simulink model "fsm_12B_global"  (R2024b)
settings: Solver=FixedStepAuto  StartTime=0.0  StopTime=10  RelTol=1e-3
settings Model: Creator=elliocm  LastModifiedBy=lukeubun
settings SolverCC: AlgebraicLoopSolver=TrustRegion
settings DataIOCC: LimitDataPoints=on  SaveFormat=Array  ReturnWorkspaceOutputs=off
settings OptimizationCC: DefaultParameterBehavior=Inlined  UseDivisionForNetSlopeComputation=on  GainParamInheritBuiltInType=on  UseFloatMulNetSlope=on  InlineInvariantSignals=on  PassReuseOutputArgsAs=Individual arguments  ExpressionDepthLimit=2147483647  ZeroExternalMemoryAtStartup=off  ZeroInternalMemoryAtStartup=off  NoFixptDivByZeroProtection=on  EfficientFloat2IntCast=on  LifeSpan=1  OptimizeBlockOrder=speed  DifferentSizesBufferReuse=on  EfficientTunableParamExpr=on
settings DebuggingCC: UnderspecifiedInitializationDetection=Classic  MergeDetectMultiDrivingBlocksExec=none  SolverPrmCheckMsg=warning  ParameterTunabilityLossMsg=error  UnconnectedInputMsg=warning  UnconnectedOutputMsg=warning  UnconnectedLineMsg=warning  StateNameClashWarn=warning  SFUnexpectedBacktrackingDiag=warning  SFNoUnconditionalDefaultTransitionDiag=warning  SFExecutionAtInitializationDiag=none  ArithmeticOperatorsInVariantConditions=warning
settings HardwareCC: ProdBitPerPointer=32  ProdBitPerSizeT=32  ProdBitPerPtrDiffT=32  ProdLargestAtomicInteger=Long  ProdWordSize=32  ProdLongLongMode=on  ProdHWDeviceType=ARM Compatible->ARM 10
settings ModelReferenceCC: PropagateSignalLabelsOutOfModel=off
settings SFSimCC: SimUseLocalCustomCode=off  MATLABDynamicMemAlloc=off  CustomCodeUndefinedFunction=UseInterfaceOnly
settings RTWCC: Description=Embedded Coder  SystemTargetFile=ert.tlc  TemplateMakefile=ert_default_tmf  RTWUseLocalCustomCode=off  GPUComputeCapability=3.5
settings CodeAppCC: ForceParamTrailComments=on  IgnoreCustomStorageClasses=off  OperatorAnnotations=on  SimulinkDataObjDesc=on  SFDataObjDesc=on  CustomSymbolStrGlobalVar=rt$N$M  CustomSymbolStrType=$N$M  CustomSymbolStrFcn=$N$M$F  CustomSymbolStrMacro=$N$M  InsertBlockDesc=on
settings ERTTargetCC: GenerateSampleERTMain=on  IncludeMdlTerminateFcn=off  CombineSignalStateStructs=on  SupportAbsoluteTime=off  SupportComplex=off  SupportContinuousTime=on  ERTCustomFileTemplate=example_file_process.tlc  ERTFilePackagingFormat=CompactWithDataFile
settings ConfigComp: CovMetricSettings=dw  CovSaveCumulativeToWorkspaceVar=on  CovSaveSingleToWorkspaceVar=on  CovExternalEMLEnable=off

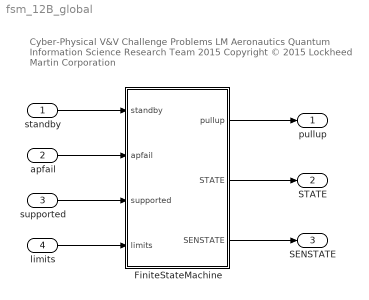
== system fsm_12B_global ==
  note: Cyber-Physical V&V Challenge Problems
      | LM Aeronautics Quantum Information Science Research Team 2015
      | Copyright © 2015 Lockheed Martin Corporation
  standby : Inport  OutDataTypeStr=boolean
  apfail : Inport  Port=2  OutDataTypeStr=boolean
  supported : Inport  Port=3  OutDataTypeStr=boolean
  limits : Inport  Port=4  OutDataTypeStr=boolean
  FiniteStateMachine : Subsystem
  pullup : Outport
  STATE : Outport  Port=2
  SENSTATE : Outport  Port=3
  wires:
  standby/1 -> FiniteStateMachine/1(standby)
  apfail/1 -> FiniteStateMachine/2(apfail)
  supported/1 -> FiniteStateMachine/3(supported)
  limits/1 -> FiniteStateMachine/4(limits)
  FiniteStateMachine/1(pullup) -> pullup/1
  FiniteStateMachine/2(STATE) -> STATE/1
  FiniteStateMachine/3(SENSTATE) -> SENSTATE/1

== system fsm_12B_global/FiniteStateMachine ==
  note: 51
  standby : Inport
  apfail : Inport  Port=2
  supported : Inport  Port=3
  limits : Inport  Port=4
  Manager : Subsystem
  Sen : Subsystem
  Unit Delay : UnitDelay  SampleTime=-1  HasFrameUpgradeWarning=on
  Unit Delay1 : UnitDelay  SampleTime=-1  HasFrameUpgradeWarning=on
  Unit Delay2 : UnitDelay  InitialCondition=1  SampleTime=-1  HasFrameUpgradeWarning=on
  pullup : Outport
  STATE : Outport  Port=2
  SENSTATE : Outport  Port=3
  wires:
  Manager/1(MODE) -> Sen/1(mode)
  Manager/4(STATE) -> Unit Delay/1, STATE/1
  Unit Delay/1 -> Manager/5(state)
  Manager/2(REQUEST) -> Sen/2(request)
  Unit Delay1/1 -> Sen/4(senstate)
  Unit Delay2/1 -> Manager/4(good)
  Sen/2(SENSTATE) -> SENSTATE/1, Unit Delay1/1
  Sen/1(good) -> Unit Delay2/1
  Manager/3(PULL) -> pullup/1
  standby/1 -> Manager/1(standby)
  apfail/1 -> Manager/2(apfail)
  supported/1 -> Manager/3(supported)
  limits/1 -> Sen/3(limits)

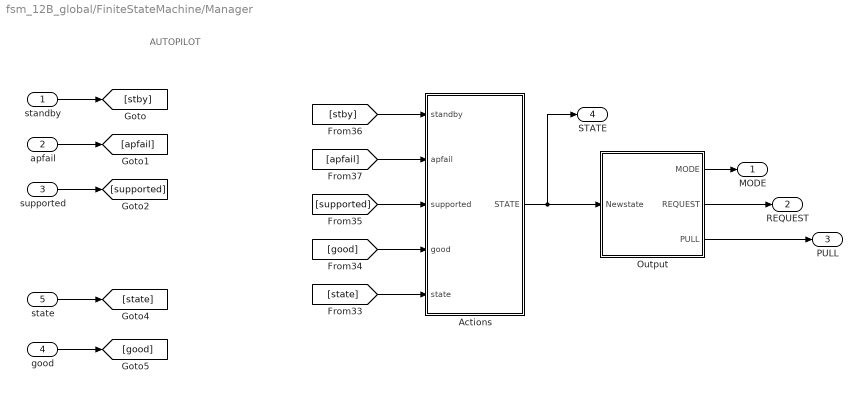
== system fsm_12B_global/FiniteStateMachine/Manager ==
  note: AUTOPILOT
  standby : Inport
  apfail : Inport  Port=2
  supported : Inport  Port=3
  good : Inport  Port=4
  state : Inport  Port=5
  Actions : Subsystem
  Output : Subsystem
  MODE : Outport
  REQUEST : Outport  Port=2
  PULL : Outport  Port=3
  STATE : Outport  Port=4
  wires:
  standby/1 -> [stby]
  supported/1 -> [supported]
  apfail/1 -> [apfail]
  state/1 -> [state]
  good/1 -> [good]
  Actions/1(STATE) -> STATE/1, Output/1(Newstate)
  [apfail] -> Actions/2(apfail)
  [state] -> Actions/5(state)
  [supported] -> Actions/3(supported)
  [good] -> Actions/4(good)
  [stby] -> Actions/1(standby)
  Output/1(MODE) -> MODE/1
  Output/2(REQUEST) -> REQUEST/1
  Output/3(PULL) -> PULL/1

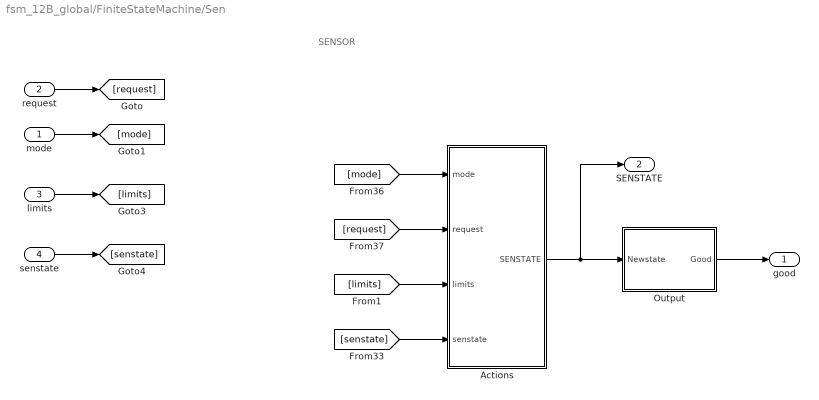
== system fsm_12B_global/FiniteStateMachine/Sen ==
  note: SENSOR
  mode : Inport
  request : Inport  Port=2
  limits : Inport  Port=3
  senstate : Inport  Port=4
  Actions : Subsystem
  Output : Subsystem
  good : Outport
  SENSTATE : Outport  Port=2
  wires:
  request/1 -> [request]
  mode/1 -> [mode]
  limits/1 -> [limits]
  senstate/1 -> [senstate]
  Output/1(Good) -> good/1
  [request] -> Actions/2(request)
  [mode] -> Actions/1(mode)
  Actions/1(SENSTATE) -> Output/1(Newstate), SENSTATE/1
  [senstate] -> Actions/4(senstate)
  [limits] -> Actions/3(limits)

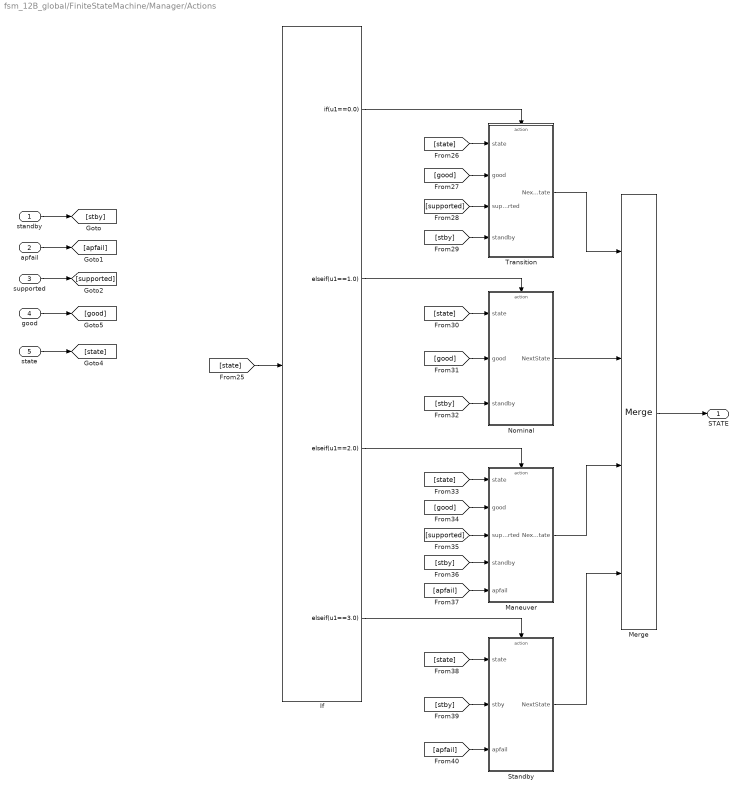
== system fsm_12B_global/FiniteStateMachine/Manager/Actions ==
  standby : Inport
  apfail : Inport  Port=2
  supported : Inport  Port=3
  good : Inport  Port=4
  state : Inport  Port=5
  If : If  IfExpression=u1==0.0  ElseIfExpressions=u1==1.0, u1==2.0, u1==3.0  ShowElse=off
  Maneuver : Subsystem
  Merge : Merge  Inputs=4
  Nominal : Subsystem
  Standby : Subsystem
  Transition : Subsystem
  STATE : Outport
  wires:
  [state] -> If/1
  [state] -> Transition/1(state)
  [apfail] -> Standby/3(apfail)
  [stby] -> Standby/2(stby)
  Standby/1(NextState) -> Merge/4
  [state] -> Standby/1(state)
  Maneuver/1(NextState) -> Merge/3
  Merge/1 -> STATE/1
  Transition/1(NextState) -> Merge/1
  Nominal/1(NextState) -> Merge/2
  If/2 -> Nominal/Action
  [state] -> Nominal/1(state)
  If/3 -> Maneuver/Action
  If/4 -> Standby/Action
  [apfail] -> Maneuver/5(apfail)
  [good] -> Nominal/2(good)
  [stby] -> Nominal/3(standby)
  If/1 -> Transition/Action
  [supported] -> Transition/3(supported)
  [good] -> Transition/2(good)
  [stby] -> Transition/4(standby)
  [state] -> Maneuver/1(state)
  [supported] -> Maneuver/3(supported)
  [good] -> Maneuver/2(good)
  [stby] -> Maneuver/4(standby)
  standby/1 -> [stby]
  supported/1 -> [supported]
  apfail/1 -> [apfail]
  state/1 -> [state]
  good/1 -> [good]

== system fsm_12B_global/FiniteStateMachine/Manager/Output ==
  Newstate : Inport
  Demux : Demux  Outputs=3
  If : If  IfExpression=u1==0.0  ElseIfExpressions=u1==1.0, u1==2.0, u1==3.0  ShowElse=off
  Maneuver : Subsystem
  Merge : Merge  Inputs=4
  Nominal : Subsystem
  Standby : Subsystem
  Transition : Subsystem
  MODE : Outport
  REQUEST : Outport  Port=2
  PULL : Outport  Port=3
  wires:
  Demux/2 -> REQUEST/1  "REQUEST"
  Demux/1 -> MODE/1  "MODE"
  Demux/3 -> PULL/1  "PULL"
  Merge/1 -> Demux/1
  Nominal/1(Output) -> Merge/2
  Maneuver/1(Output) -> Merge/3
  If/2 -> Nominal/Action
  Transition/1(Output) -> Merge/1
  If/3 -> Maneuver/Action
  Standby/1(Output) -> Merge/4
  If/1 -> Transition/Action
  Newstate/1 -> If/1
  If/4 -> Standby/Action

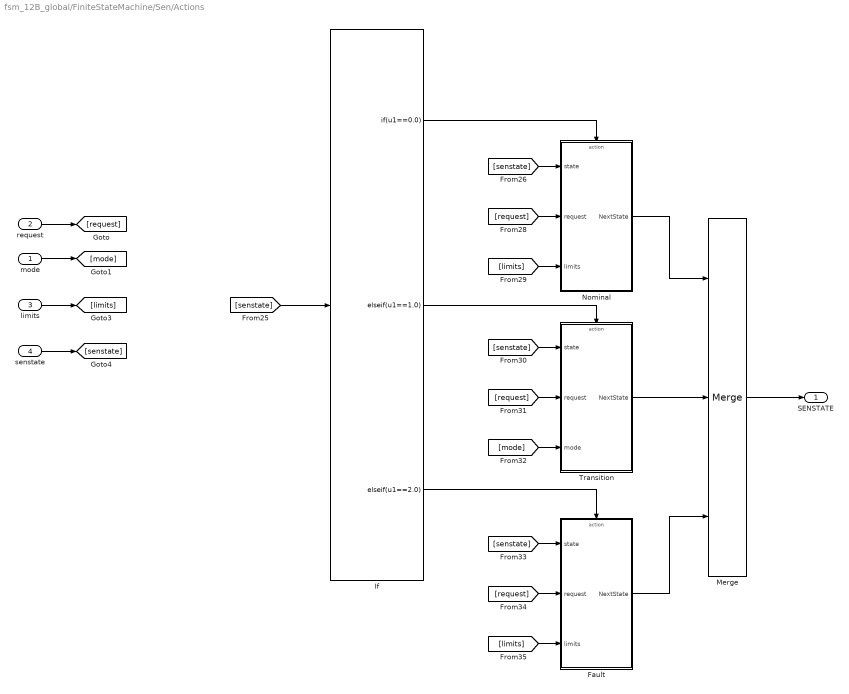
== system fsm_12B_global/FiniteStateMachine/Sen/Actions ==
  mode : Inport
  request : Inport  Port=2
  limits : Inport  Port=3
  senstate : Inport  Port=4
  Fault : Subsystem
  If : If  IfExpression=u1==0.0  ElseIfExpressions=u1==1.0, u1==2.0  ShowElse=off
  Merge : Merge  Inputs=3
  Nominal : Subsystem
  Transition : Subsystem
  SENSTATE : Outport
  wires:
  [senstate] -> If/1
  [senstate] -> Nominal/1(state)
  Fault/1(NextState) -> Merge/3
  Merge/1 -> SENSTATE/1
  Nominal/1(NextState) -> Merge/1
  Transition/1(NextState) -> Merge/2
  If/2 -> Transition/Action
  [senstate] -> Transition/1(state)
  If/3 -> Fault/Action
  [request] -> Transition/2(request)
  [mode] -> Transition/3(mode)
  If/1 -> Nominal/Action
  [request] -> Nominal/2(request)
  [limits] -> Nominal/3(limits)
  [senstate] -> Fault/1(state)
  [limits] -> Fault/3(limits)
  [request] -> Fault/2(request)
  request/1 -> [request]
  mode/1 -> [mode]
  limits/1 -> [limits]
  senstate/1 -> [senstate]

== system fsm_12B_global/FiniteStateMachine/Sen/Output ==
  Newstate : Inport
  Constant12 : Constant  OutDataTypeStr=boolean
  Constant6 : Constant  Value=2
  Constant9 : Constant  Value=0  OutDataTypeStr=boolean
  Relational Operator5 : RelationalOperator  Operator===  OutDataTypeStr=boolean  InputSameDT=off
  Switch2 : Switch  Criteria=u2 ~= 0  SaturateOnIntegerOverflow=off  InputSameDT=off
  Good : Outport
  wires:
  Constant6/1 -> Relational Operator5/2
  Relational Operator5/1 -> Switch2/2
  Constant9/1 -> Switch2/1
  Constant12/1 -> Switch2/3
  Switch2/1 -> Good/1
  Newstate/1 -> Relational Operator5/1

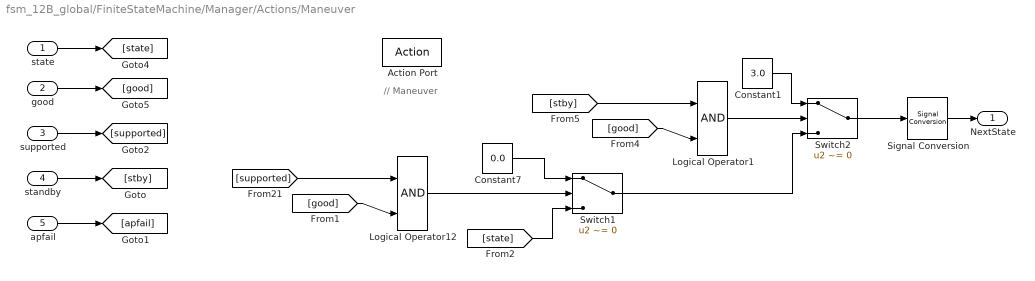
== system fsm_12B_global/FiniteStateMachine/Manager/Actions/Maneuver ==
  note: // Maneuver
  state : Inport
  good : Inport  Port=2
  supported : Inport  Port=3
  standby : Inport  Port=4
  apfail : Inport  Port=5
  Action Port : ActionPort  ActionPortLabel=elseif( u1==2.0)
  Constant1 : Constant  Value=3.0
  Constant7 : Constant  Value=0.0
  Logical Operator1 : Logic  IconShape=distinctive  AllPortsSameDT=off  OutDataTypeStr=boolean
  Logical Operator12 : Logic  IconShape=distinctive  AllPortsSameDT=off  OutDataTypeStr=boolean
  Signal Conversion : SignalConversion  OverrideOpt=off
  Switch1 : Switch  Criteria=u2 ~= 0  SaturateOnIntegerOverflow=off  InputSameDT=off
  Switch2 : Switch  Criteria=u2 ~= 0  SaturateOnIntegerOverflow=off  InputSameDT=off
  NextState : Outport
  wires:
  [supported] -> Logical Operator12/1
  Logical Operator12/1 -> Switch1/2
  [state] -> Switch1/3
  Constant7/1 -> Switch1/1
  Logical Operator1/1 -> Switch2/2
  Constant1/1 -> Switch2/1
  Switch2/1 -> Signal Conversion/1
  Signal Conversion/1 -> NextState/1
  standby/1 -> [stby]
  supported/1 -> [supported]
  apfail/1 -> [apfail]
  state/1 -> [state]
  good/1 -> [good]
  [good] -> Logical Operator12/2
  [stby] -> Logical Operator1/1
  [good] -> Logical Operator1/2
  Switch1/1 -> Switch2/3

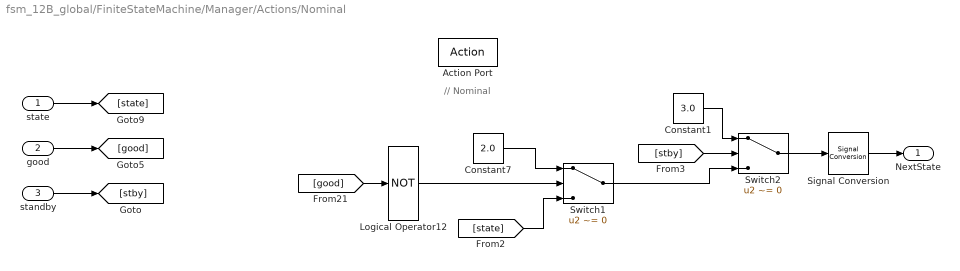
== system fsm_12B_global/FiniteStateMachine/Manager/Actions/Nominal ==
  note: // Nominal
  state : Inport
  good : Inport  Port=2
  standby : Inport  Port=3
  Action Port : ActionPort  ActionPortLabel=elseif(u1==1.0)
  Constant1 : Constant  Value=3.0
  Constant7 : Constant  Value=2.0
  Logical Operator12 : Logic  Operator=NOT  IconShape=distinctive  AllPortsSameDT=off  OutDataTypeStr=boolean
  Signal Conversion : SignalConversion  OverrideOpt=off
  Switch1 : Switch  Criteria=u2 ~= 0  SaturateOnIntegerOverflow=off  InputSameDT=off
  Switch2 : Switch  Criteria=u2 ~= 0  SaturateOnIntegerOverflow=off  InputSameDT=off
  NextState : Outport
  wires:
  Signal Conversion/1 -> NextState/1
  Switch2/1 -> Signal Conversion/1
  Switch1/1 -> Switch2/3
  Constant1/1 -> Switch2/1
  [stby] -> Switch2/2
  standby/1 -> [stby]
  Constant7/1 -> Switch1/1
  [state] -> Switch1/3
  Logical Operator12/1 -> Switch1/2
  [good] -> Logical Operator12/1
  good/1 -> [good]
  state/1 -> [state]

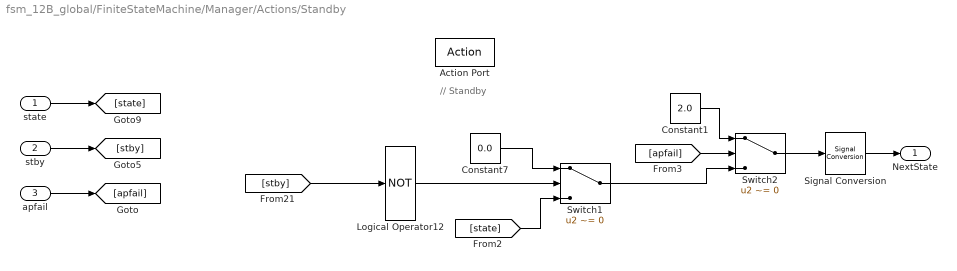
== system fsm_12B_global/FiniteStateMachine/Manager/Actions/Standby ==
  note: // Standby
  state : Inport
  stby : Inport  Port=2
  apfail : Inport  Port=3
  Action Port : ActionPort  ActionPortLabel=elseif( u1==3.0)
  Constant1 : Constant  Value=2.0
  Constant7 : Constant  Value=0.0
  Logical Operator12 : Logic  Operator=NOT  IconShape=distinctive  AllPortsSameDT=off  OutDataTypeStr=boolean
  Signal Conversion : SignalConversion  OverrideOpt=off
  Switch1 : Switch  Criteria=u2 ~= 0  SaturateOnIntegerOverflow=off  InputSameDT=off
  Switch2 : Switch  Criteria=u2 ~= 0  SaturateOnIntegerOverflow=off  InputSameDT=off
  NextState : Outport
  wires:
  Signal Conversion/1 -> NextState/1
  Switch2/1 -> Signal Conversion/1
  Switch1/1 -> Switch2/3
  Constant1/1 -> Switch2/1
  [apfail] -> Switch2/2
  apfail/1 -> [apfail]
  Constant7/1 -> Switch1/1
  [state] -> Switch1/3
  Logical Operator12/1 -> Switch1/2
  [stby] -> Logical Operator12/1
  stby/1 -> [stby]
  state/1 -> [state]

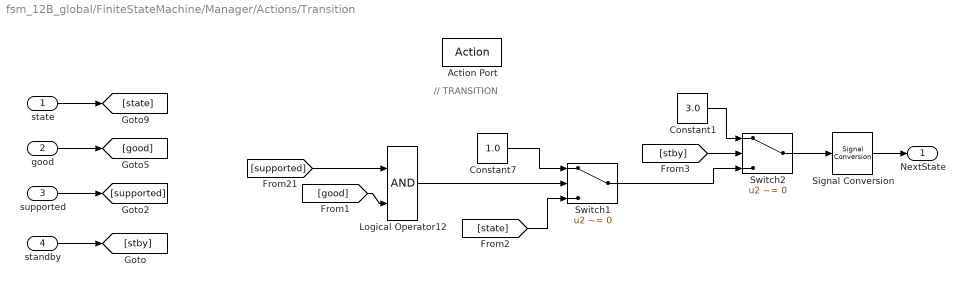
== system fsm_12B_global/FiniteStateMachine/Manager/Actions/Transition ==
  note: // TRANSITION
  state : Inport
  good : Inport  Port=2
  supported : Inport  Port=3
  standby : Inport  Port=4
  Action Port : ActionPort  ActionPortLabel=if(u1==0.0)
  Constant1 : Constant  Value=3.0
  Constant7 : Constant  Value=1.0
  Logical Operator12 : Logic  IconShape=distinctive  AllPortsSameDT=off  OutDataTypeStr=boolean
  Signal Conversion : SignalConversion  OverrideOpt=off
  Switch1 : Switch  Criteria=u2 ~= 0  SaturateOnIntegerOverflow=off  InputSameDT=off
  Switch2 : Switch  Criteria=u2 ~= 0  SaturateOnIntegerOverflow=off  InputSameDT=off
  NextState : Outport
  wires:
  state/1 -> [state]
  good/1 -> [good]
  supported/1 -> [supported]
  [supported] -> Logical Operator12/1
  [good] -> Logical Operator12/2
  Logical Operator12/1 -> Switch1/2
  [state] -> Switch1/3
  Constant7/1 -> Switch1/1
  standby/1 -> [stby]
  [stby] -> Switch2/2
  Constant1/1 -> Switch2/1
  Switch1/1 -> Switch2/3
  Switch2/1 -> Signal Conversion/1
  Signal Conversion/1 -> NextState/1

== system fsm_12B_global/FiniteStateMachine/Manager/Output/Maneuver ==
  note: // Maneuver
  note: PULL
  Action Port : ActionPort  ActionPortLabel=elseif( u1==2.0)
  Constant10 : Constant  OutDataTypeStr=boolean
  Constant11 : Constant  OutDataTypeStr=boolean
  Constant9 : Constant  OutDataTypeStr=boolean
  Mux2 : Mux  Inputs=3
  Output : Outport
  wires:
  Mux2/1 -> Output/1
  Constant10/1 -> Mux2/2
  Constant11/1 -> Mux2/3
  Constant9/1 -> Mux2/1

== system fsm_12B_global/FiniteStateMachine/Manager/Output/Nominal ==
  note: // Nominal
  note: OPS
  Action Port : ActionPort  ActionPortLabel=elseif(u1==1.0)
  Constant3 : Constant  OutDataTypeStr=boolean
  Constant4 : Constant  OutDataTypeStr=boolean
  Constant5 : Constant  Value=0  OutDataTypeStr=boolean
  Mux1 : Mux  Inputs=3
  Output : Outport
  wires:
  Constant5/1 -> Mux1/3
  Constant4/1 -> Mux1/2
  Constant3/1 -> Mux1/1
  Mux1/1 -> Output/1

== system fsm_12B_global/FiniteStateMachine/Manager/Output/Standby ==
  note: PULL
  note: // Standby
  Action Port : ActionPort  ActionPortLabel=elseif( u1==3.0)
  Constant1 : Constant  Value=0  OutDataTypeStr=boolean
  Constant11 : Constant  Value=0  OutDataTypeStr=boolean
  Constant9 : Constant  OutDataTypeStr=boolean
  Mux2 : Mux  Inputs=3
  Output : Outport
  wires:
  Constant9/1 -> Mux2/1
  Constant11/1 -> Mux2/3
  Constant1/1 -> Mux2/2
  Mux2/1 -> Output/1

== system fsm_12B_global/FiniteStateMachine/Manager/Output/Transition ==
  note: // TRANSITION
  note: TRANSITION
  Action Port : ActionPort  ActionPortLabel=if(u1==0.0)
  Constant16 : Constant  Value=0  OutDataTypeStr=boolean
  Constant17 : Constant  OutDataTypeStr=boolean
  Constant18 : Constant  Value=0  OutDataTypeStr=boolean
  Mux4 : Mux  Inputs=3
  Output : Outport
  wires:
  Mux4/1 -> Output/1
  Constant17/1 -> Mux4/2
  Constant16/1 -> Mux4/1
  Constant18/1 -> Mux4/3

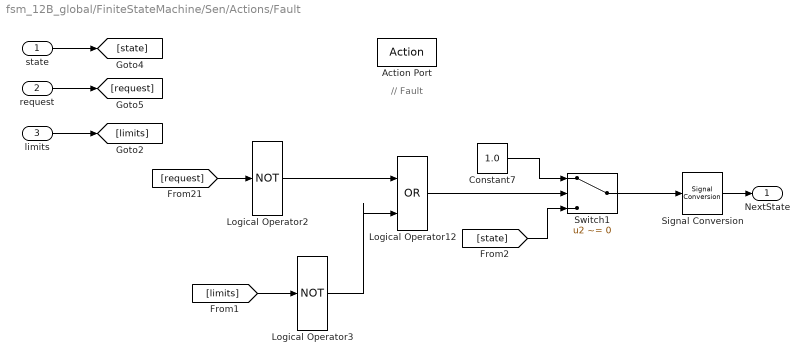
== system fsm_12B_global/FiniteStateMachine/Sen/Actions/Fault ==
  note: // Fault
  state : Inport
  request : Inport  Port=2
  limits : Inport  Port=3
  Action Port : ActionPort  ActionPortLabel=elseif( u1==2.0)
  Constant7 : Constant  Value=1.0
  Logical Operator12 : Logic  Operator=OR  IconShape=distinctive  AllPortsSameDT=off  OutDataTypeStr=boolean
  Logical Operator2 : Logic  Operator=NOT  IconShape=distinctive  AllPortsSameDT=off  OutDataTypeStr=boolean
  Logical Operator3 : Logic  Operator=NOT  IconShape=distinctive  AllPortsSameDT=off  OutDataTypeStr=boolean
  Signal Conversion : SignalConversion  OverrideOpt=off
  Switch1 : Switch  Criteria=u2 ~= 0  SaturateOnIntegerOverflow=off  InputSameDT=off
  NextState : Outport
  wires:
  [request] -> Logical Operator2/1
  Logical Operator12/1 -> Switch1/2
  [state] -> Switch1/3
  Constant7/1 -> Switch1/1
  Switch1/1 -> Signal Conversion/1
  Signal Conversion/1 -> NextState/1
  limits/1 -> [limits]
  state/1 -> [state]
  request/1 -> [request]
  Logical Operator2/1 -> Logical Operator12/1
  [limits] -> Logical Operator3/1
  Logical Operator3/1 -> Logical Operator12/2

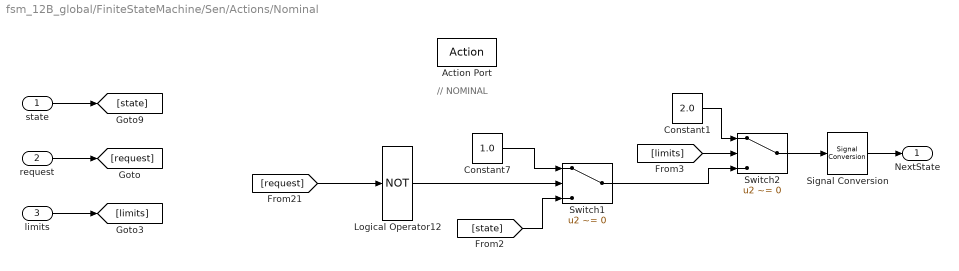
== system fsm_12B_global/FiniteStateMachine/Sen/Actions/Nominal ==
  note: // NOMINAL
  state : Inport
  request : Inport  Port=2
  limits : Inport  Port=3
  Action Port : ActionPort  ActionPortLabel=if(u1==0.0)
  Constant1 : Constant  Value=2.0
  Constant7 : Constant  Value=1.0
  Logical Operator12 : Logic  Operator=NOT  IconShape=distinctive  AllPortsSameDT=off  OutDataTypeStr=boolean
  Signal Conversion : SignalConversion  OverrideOpt=off
  Switch1 : Switch  Criteria=u2 ~= 0  SaturateOnIntegerOverflow=off  InputSameDT=off
  Switch2 : Switch  Criteria=u2 ~= 0  SaturateOnIntegerOverflow=off  InputSameDT=off
  NextState : Outport
  wires:
  state/1 -> [state]
  [request] -> Logical Operator12/1
  Logical Operator12/1 -> Switch1/2
  [state] -> Switch1/3
  Constant7/1 -> Switch1/1
  [limits] -> Switch2/2
  Constant1/1 -> Switch2/1
  Switch1/1 -> Switch2/3
  Switch2/1 -> Signal Conversion/1
  Signal Conversion/1 -> NextState/1
  request/1 -> [request]
  limits/1 -> [limits]

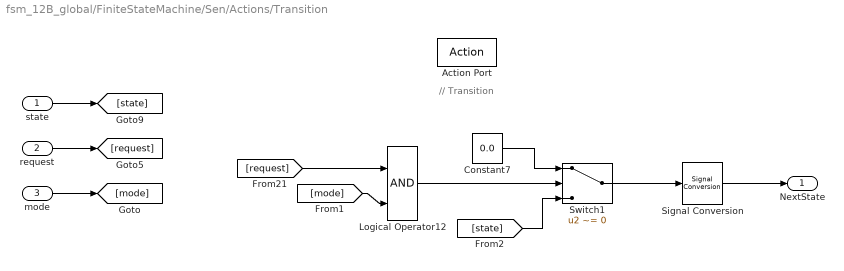
== system fsm_12B_global/FiniteStateMachine/Sen/Actions/Transition ==
  note: // Transition
  state : Inport
  request : Inport  Port=2
  mode : Inport  Port=3
  Action Port : ActionPort  ActionPortLabel=elseif(u1==1.0)
  Constant7 : Constant  Value=0.0
  Logical Operator12 : Logic  IconShape=distinctive  AllPortsSameDT=off  OutDataTypeStr=boolean
  Signal Conversion : SignalConversion  OverrideOpt=off
  Switch1 : Switch  Criteria=u2 ~= 0  SaturateOnIntegerOverflow=off  InputSameDT=off
  NextState : Outport
  wires:
  Signal Conversion/1 -> NextState/1
  Switch1/1 -> Signal Conversion/1
  mode/1 -> [mode]
  Constant7/1 -> Switch1/1
  [state] -> Switch1/3
  Logical Operator12/1 -> Switch1/2
  [request] -> Logical Operator12/1
  request/1 -> [request]
  state/1 -> [state]
  [mode] -> Logical Operator12/2
